simulink model "quad_modified"  (Simulink 7.8)
settings: Solver=ode45  StartTime=0.0  StopTime=10.0  RelTol=1e-3
InitFcn:
  | % load parameters of the default quadrotor
  | disp('Quadrotor parameters loaded by InitFcn')
  | mdl_quadcopter
undefined symbols (not defined in the file or in its folder): quad
libraries: roblocks x3, simulink x1
settings Model: Creator=deep  LastModifiedBy=deep

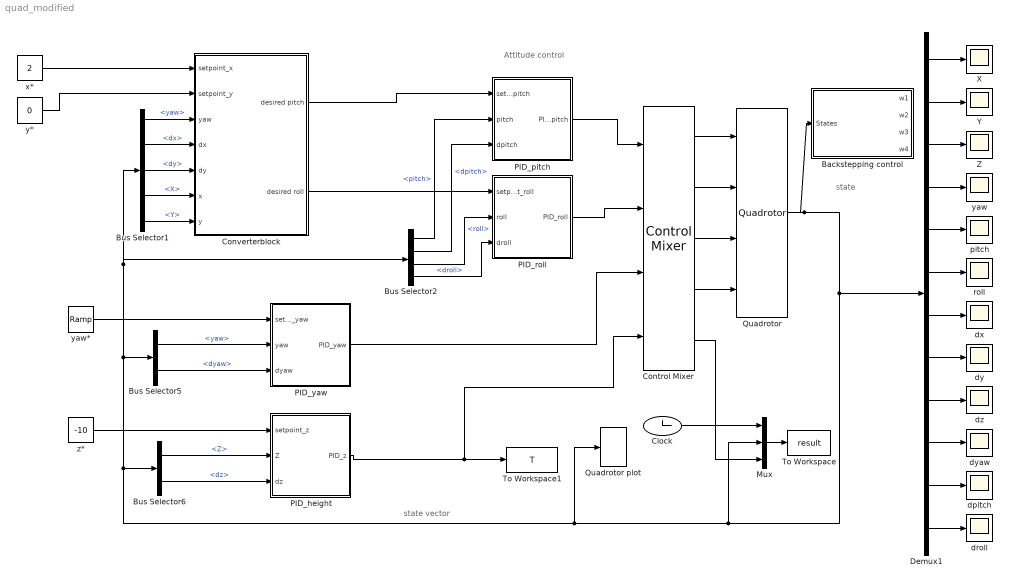
== system quad_modified ==
  note: state vector
  note: state
  note: Attitude control
  Backstepping control : Subsystem  AncestorBlock=roblocks/Dynamics/Control Mixer
  Bus Selector1 : BusSelector  OutputSignals=yaw,dx,dy,X,Y
  Bus Selector2 : BusSelector  OutputSignals=pitch,dpitch,roll,droll
  Bus Selector5 : BusSelector  OutputSignals=yaw,dyaw
  Bus Selector6 : BusSelector  OutputSignals=Z,dz
  Clock : Clock
  Control Mixer : roblocks/Dynamics/Control Mixer
      link override Saturation1: UpperLimit=1000
      link override Saturation2: UpperLimit=1000
      link override Saturation3: UpperLimit=1000
      link override Saturation4: UpperLimit=1000
  Converterblock : Subsystem  AncestorBlock=roblocks/Dynamics/Control Mixer
  Demux1 : Demux  Outputs=12  BusSelectionMode=on
  Mux : Mux  Inputs=3
  PID_height : Subsystem  AncestorBlock=roblocks/Dynamics/Control Mixer
  PID_pitch : Subsystem  AncestorBlock=roblocks/Dynamics/Control Mixer
  PID_roll : Subsystem  AncestorBlock=roblocks/Dynamics/Control Mixer
  PID_yaw : Subsystem  AncestorBlock=roblocks/Dynamics/Control Mixer
  Quadrotor : roblocks/Dynamics/Quadrotor
  Quadrotor plot : roblocks/Robot Graphics/Quadrotor plot
      link override Plotter: Parameters=[2,10], 1, 1
  To Workspace : ToWorkspace  VariableName=result  SampleTime=-1  SaveFormat=Array
  To Workspace1 : ToWorkspace  VariableName=T  SampleTime=-1  SaveFormat=Array
  X : Scope
      settings: YMin=-0.04  YMax=0.045
  Y : Scope
      settings: YMin=-0.04  YMax=0.045  SaveName=ScopeData2
  Z : Scope
      settings: YMin=-0.04  YMax=0.045  SaveName=ScopeData3
  dpitch : Scope
      settings: YMin=-0.04  YMax=0.045  SaveName=ScopeData11
  droll : Scope
      settings: YMin=-0.04  YMax=0.045  SaveName=ScopeData12
  dx : Scope
      settings: YMin=-0.04  YMax=0.045  SaveName=ScopeData7
  dy : Scope
      settings: YMin=-0.04  YMax=0.045  SaveName=ScopeData8
  dyaw : Scope
      settings: YMin=-0.04  YMax=0.045  SaveName=ScopeData10
  dz : Scope
      settings: YMin=-0.04  YMax=0.045  SaveName=ScopeData9
  pitch : Scope
      settings: YMin=-0.04  YMax=0.045  SaveName=ScopeData5
  roll : Scope
      settings: YMin=-0.04  YMax=0.045  SaveName=ScopeData6
  x* : Constant  Value=2
  y* : Constant  Value=0
  yaw : Scope
      settings: YMin=-0.04  YMax=0.045  SaveName=ScopeData4
  yaw* : simulink/Sources/Ramp  slope=0  start=0  X0=0
  z* : Constant  Value=-10  SampleTime=0
  wires:
  Control Mixer/1 -> Quadrotor/1
  Control Mixer/4 -> Quadrotor/4
  Quadrotor/1 -> Bus Selector6/1, Bus Selector5/1, Bus Selector1/1, Bus Selector2/1, Quadrotor plot/1, Mux/2, Demux1/1, Backstepping control/1(States)
  PID_yaw/1(PID_yaw) -> Control Mixer/3
  Bus Selector5/1 -> PID_yaw/2(yaw)  "<yaw>"
  z*/1 -> PID_height/1(setpoint_z)
  Mux/1 -> To Workspace/1
  Clock/1 -> Mux/1
  Control Mixer/5 -> Mux/3
  Control Mixer/3 -> Quadrotor/3
  Control Mixer/2 -> Quadrotor/2
  Demux1/1 -> X/1
  Demux1/2 -> Y/1
  Demux1/3 -> Z/1
  Demux1/4 -> yaw/1
  Demux1/5 -> pitch/1
  Demux1/6 -> roll/1
  Demux1/7 -> dx/1
  Demux1/8 -> dy/1
  Demux1/9 -> dz/1
  Demux1/10 -> dyaw/1
  Demux1/11 -> dpitch/1
  Demux1/12 -> droll/1
  Bus Selector6/1 -> PID_height/2(Z)  "<Z>"
  Bus Selector6/2 -> PID_height/3(dz)  "<dz>"
  PID_height/1(PID_z) -> Control Mixer/4, To Workspace1/1
  yaw*/1 -> PID_yaw/1(setpoint_yaw)
  Bus Selector5/2 -> PID_yaw/3(dyaw)  "<dyaw>"
  x*/1 -> Converterblock/1(setpoint_x)
  y*/1 -> Converterblock/2(setpoint_y)
  Bus Selector1/2 -> Converterblock/4(dx)  "<dx>"
  Bus Selector1/1 -> Converterblock/3(yaw)  "<yaw>"
  Bus Selector1/3 -> Converterblock/5(dy)  "<dy>"
  Bus Selector1/4 -> Converterblock/6(x)  "<X>"
  Bus Selector1/5 -> Converterblock/7(y)  "<Y>"
  PID_pitch/1(PID_pitch) -> Control Mixer/1
  PID_roll/1(PID_roll) -> Control Mixer/2
  Converterblock/1(desired pitch) -> PID_pitch/1(setpoint_pitch)
  Converterblock/2(desired roll) -> PID_roll/1(setpoint_roll)
  Bus Selector2/1 -> PID_pitch/2(pitch)  "<pitch>"
  Bus Selector2/2 -> PID_pitch/3(dpitch)  "<dpitch>"
  Bus Selector2/3 -> PID_roll/2(roll)  "<roll>"
  Bus Selector2/4 -> PID_roll/3(droll)  "<droll>"

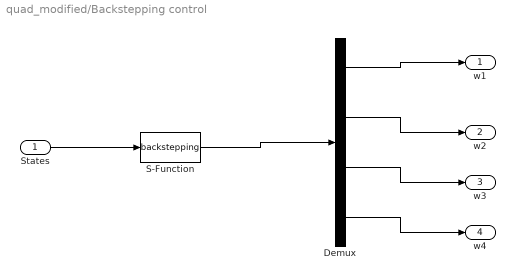
== system quad_modified/Backstepping control ==
  States : Inport
  Demux : Demux
  S-Function : S-Function  FunctionName=backstepping  Parameters=quad  EnableBusSupport=off
  w1 : Outport
  w2 : Outport  Port=2
  w3 : Outport  Port=3
  w4 : Outport  Port=4
  wires:
  States/1 -> S-Function/1
  Demux/1 -> w1/1
  Demux/2 -> w2/1
  Demux/3 -> w3/1
  Demux/4 -> w4/1
  S-Function/1 -> Demux/1

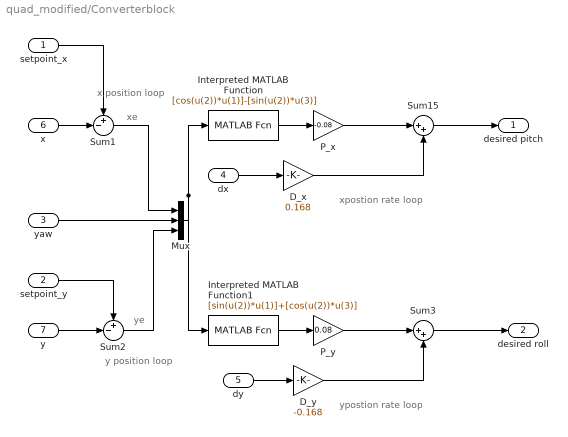
== system quad_modified/Converterblock ==
  note: xpostion rate
      | loop
  note: x position
      | loop
  note: xe
  note: ye
  note: ypostion rate
      | loop
  note: y position loop
  setpoint_x : Inport
  setpoint_y : Inport  Port=2
  yaw : Inport  Port=3
  dx : Inport  Port=4
  dy : Inport  Port=5
  x : Inport  Port=6
  y : Inport  Port=7
  D_x : Gain  Gain=0.168
  D_y : Gain  Gain=-0.168
  Interpreted MATLAB Function : MATLABFcn  MATLABFcn=[cos(u(2))*u(1)]-[sin(u(2))*u(3)]
  Interpreted MATLAB Function1 : MATLABFcn  MATLABFcn=[sin(u(2))*u(1)]+[cos(u(2))*u(3)]
  Mux : Mux  Inputs=3
  P_x : Gain  Gain=-0.08
  P_y : Gain  Gain=0.08
  Sum1 : Sum  Inputs=+-|
  Sum15 : Sum  Inputs=|++
  Sum2 : Sum  Inputs=+-|
  Sum3 : Sum  Inputs=|++
  desired pitch : Outport
  desired roll : Outport  Port=2
  wires:
  setpoint_x/1 -> Sum1/1
  P_x/1 -> Sum15/1
  D_x/1 -> Sum15/2
  Sum15/1 -> desired pitch/1
  x/1 -> Sum1/2
  setpoint_y/1 -> Sum2/1
  y/1 -> Sum2/2
  yaw/1 -> Mux/2
  Sum1/1 -> Mux/1
  Sum2/1 -> Mux/3
  Mux/1 -> Interpreted MATLAB Function/1, Interpreted MATLAB Function1/1
  dx/1 -> D_x/1
  Interpreted MATLAB Function/1 -> P_x/1
  P_y/1 -> Sum3/1
  D_y/1 -> Sum3/2
  Sum3/1 -> desired roll/1
  dy/1 -> D_y/1
  Interpreted MATLAB Function1/1 -> P_y/1

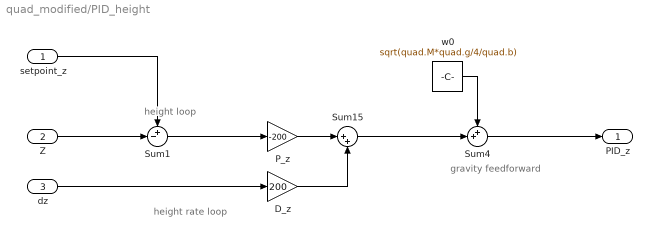
== system quad_modified/PID_height ==
  note: height rate
      | loop
  note: height
      | loop
  note: gravity feedforward
  setpoint_z : Inport
  Z : Inport  Port=2
  dz : Inport  Port=3
  D_z : Gain  Gain=200
  P_z : Gain  Gain=-200
  Sum1 : Sum  Inputs=+-|
  Sum15 : Sum  Inputs=|++
  Sum4 : Sum  Inputs=++|
  w0 : Constant  Value=sqrt(quad.M*quad.g/4/quad.b)  SampleTime=0
  PID_z : Outport
  wires:
  setpoint_z/1 -> Sum1/1
  Z/1 -> Sum1/2
  Sum1/1 -> P_z/1
  dz/1 -> D_z/1
  P_z/1 -> Sum15/1
  D_z/1 -> Sum15/2
  w0/1 -> Sum4/1
  Sum15/1 -> Sum4/2
  Sum4/1 -> PID_z/1

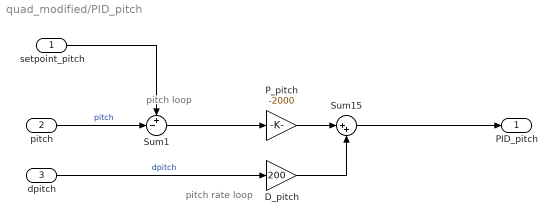
== system quad_modified/PID_pitch ==
  note: pitch rate
      | loop
  note: pitch
      | loop
  setpoint_pitch : Inport
  pitch : Inport  Port=2
  dpitch : Inport  Port=3
  D_pitch : Gain  Gain=200
  P_pitch : Gain  Gain=-2000
  Sum1 : Sum  Inputs=+-|
  Sum15 : Sum  Inputs=|++
  PID_pitch : Outport
  wires:
  setpoint_pitch/1 -> Sum1/1
  pitch/1 -> Sum1/2  "pitch"
  Sum1/1 -> P_pitch/1
  dpitch/1 -> D_pitch/1  "dpitch"
  P_pitch/1 -> Sum15/1
  D_pitch/1 -> Sum15/2
  Sum15/1 -> PID_pitch/1

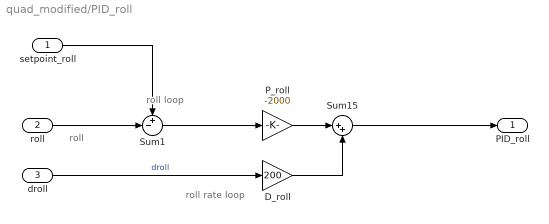
== system quad_modified/PID_roll ==
  note: roll rate
      | loop
  note: roll
      | loop
  note: roll
  setpoint_roll : Inport
  roll : Inport  Port=2
  droll : Inport  Port=3
  D_roll : Gain  Gain=200
  P_roll : Gain  Gain=-2000
  Sum1 : Sum  Inputs=+-|
  Sum15 : Sum  Inputs=|++
  PID_roll : Outport
  wires:
  setpoint_roll/1 -> Sum1/1
  roll/1 -> Sum1/2
  Sum1/1 -> P_roll/1
  droll/1 -> D_roll/1  "droll"
  P_roll/1 -> Sum15/1
  D_roll/1 -> Sum15/2
  Sum15/1 -> PID_roll/1

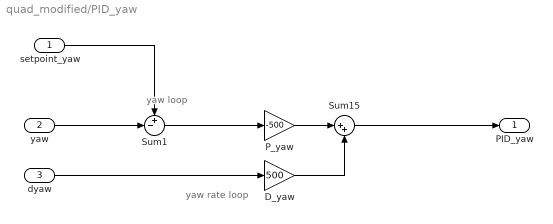
== system quad_modified/PID_yaw ==
  note: yaw rate
      | loop
  note: yaw
      | loop
  setpoint_yaw : Inport
  yaw : Inport  Port=2
  dyaw : Inport  Port=3
  D_yaw : Gain  Gain=500
  P_yaw : Gain  Gain=-500
  Sum1 : Sum  Inputs=+-|
  Sum15 : Sum  Inputs=|++
  PID_yaw : Outport
  wires:
  setpoint_yaw/1 -> Sum1/1
  yaw/1 -> Sum1/2
  Sum1/1 -> P_yaw/1
  dyaw/1 -> D_yaw/1
  P_yaw/1 -> Sum15/1
  D_yaw/1 -> Sum15/2
  Sum15/1 -> PID_yaw/1
